simulink model "my_cstr"  (R2021b)
settings: Solver=ode45  StartTime=0.0  StopTime=1600  RelTol=1e-3
libraries: slpidlib x2
settings Model: PauseTimes=1  PacingRate=1000  Creator=Yi  LastModifiedBy=admin
settings DataIOCC: ReturnWorkspaceOutputs=off

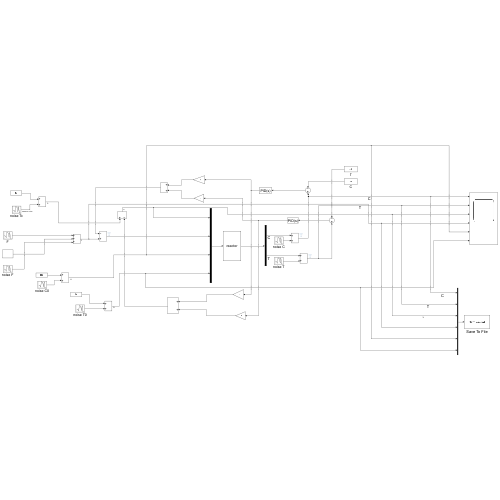
[thumbnail: Simulink's stored preview of the top-level diagram]
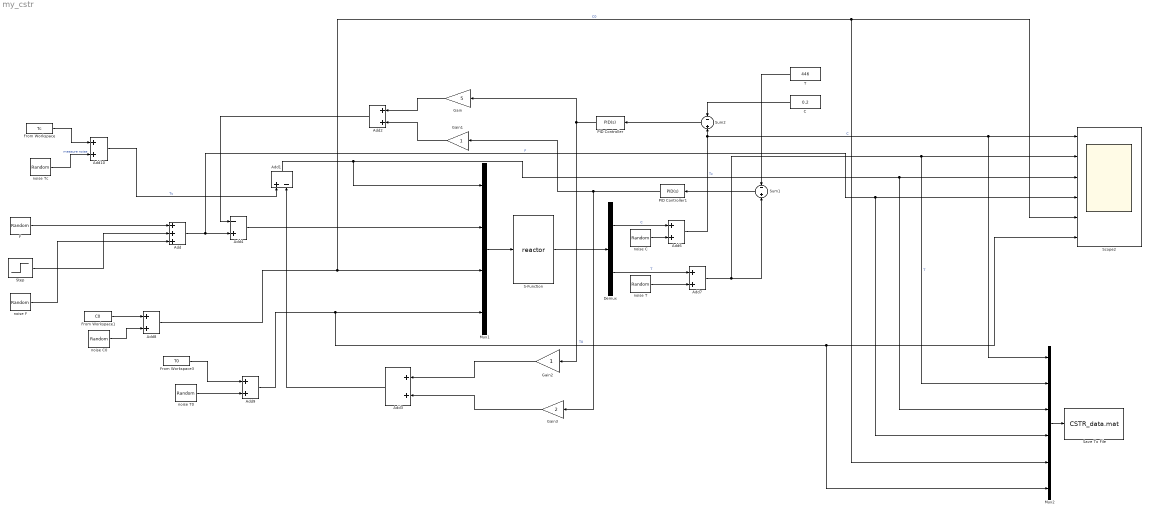
== system my_cstr ==
  Add : Sum  Inputs=+++
  Add1 : Sum  Inputs=+-
  Add{2..3,6..10} (7 alike) : Sum
  Add4 : Sum  Inputs=-+
  C : Constant  Value=0.2
  Demux : Demux  Outputs=2
  F : RandomNumber  Mean=100  Variance=30  SampleTime=1
  From Workspace : FromWorkspace  VariableName=Tc  SampleTime=1
  From Workspace1 : FromWorkspace  VariableName=C0  SampleTime=1
  From Workspace3 : FromWorkspace  VariableName=T0  SampleTime=1
  Gain : Gain  Gain=5
  Gain1 : Gain
  Gain2 : Gain
  Gain3 : Gain  Gain=2
  Mux1 : Mux
  Mux2 : Mux  Inputs=6
  PID Controller : slpidlib/PID Controller  Controller=PID  Form=Parallel  TimeDomain=Continuous-time  UseExternalTs=off  SampleTime=-1  IntegratorMethod=Forward Euler  FilterMethod=Forward Euler  ControllerParametersSource=internal  P=1  I=10  D=0.1  UseFilter=on  N=100  TunerSelectOption=Transfer Function Based (PID Tuner App)  InitialConditionSource=internal  InitialConditionForIntegrator=0  InitialConditionForFilter=0  DifferentiatorICPrevScaledInput=0  ExternalReset=none  TrackingMode=off  Kt=1  LimitOutput=off  SatLimitsSource=internal  UpperSaturationLimit=inf  LowerSaturationLimit=-inf  LinearizeAsGain=on  AntiWindupMode=none  Kb=1  POutMin=[]  POutMax=[]  IOutMin=[]  IOutMax=[]  DOutMin=[]  DOutMax=[]  NOutMin=[]  NOutMax=[]  SumOutMin=[]  SumOutMax=[]  SaturationOutMin=[]  SaturationOutMax=[]  PParamMin=[]  PParamMax=[]  IParamMin=[]  IParamMax=[]  DParamMin=[]  DParamMax=[]  NParamMin=[]  NParamMax=[]  KbParamMin=[]  KbParamMax=[]  KtParamMin=[]  KtParamMax=[]  KbOutMin=[]  KbOutMax=[]  KtOutMin=[]  KtOutMax=[]  IntegratorOutMin=[]  IntegratorOutMax=[]  FilterOutMin=[]  FilterOutMax=[]  SumI1OutMin=[]  SumI1OutMax=[]  SumI2OutMin=[]  SumI2OutMax=[]  SumI3OutMin=[]  SumI3OutMax=[]  SumI4OutMin=[]  SumI4OutMax=[]  SumDOutMin=[]  SumDOutMax=[]  DifferentiatorOutMin=[]  DifferentiatorOutMax=[]  FilterDiffOutCoefMin=[]  FilterDiffOutCoefMax=[]  ReciprocalOutMin=[]  ReciprocalOutMax=[]  SumDenOutMin=[]  SumDenOutMax=[]  SumNumOutMin=[]  SumNumOutMax=[]  DivideOutMin=[]  DivideOutMax=[]  UdiffTsProdOutMin=[]  UdiffTsProdOutMax=[]  NTsProdOutMin=[]  NTsProdOutMax=[]  UintegralTsProdOutMin=[]  UintegralTsProdOutMax=[]  UngainTsProdOutMin=[]  UngainTsProdOutMax=[]  IntegratorContinuousStateAttributes=''  IntegratorStateMustResolveToSignalObject=off  IntegratorRTWStateStorageClass=Auto  FilterContinuousStateAttributes=''  FilterStateMustResolveToSignalObject=off  FilterRTWStateStorageClass=Auto  ParallelPVariant=InternalParameters  IdealPVariant=Disabled  IVariant=InternalParameters  DVariant=InternalParameters  IntegratorVariant=Continuous  SatVariant=Disabled  AWVariant=Passthrough  PCopyVariant=Disabled  TRVariant=Disabled  FdbkBlocksVariant=Forward  IdealPFdbkVariant=Disabled  SatFdbkVariant=Disabled  DerivativeFilterVariant=ContFilter  NVariant=InternalParameters  NCopyVariant=Disabled  FilterICVariant=InternalICsFilter  IntegratorICVariant=InternalICs  ExternalResetVariant=Disabled  TRSumVariant=Passthrough  SumFdbkVariant=Disabled  SumVariant=Sum_PID  TsampFilterVariant=InternalTs  TsampNgainVariant=Passthrough  TsampIntegralVariant=Passthrough  ExternalSaturationOutDataTypeStr=Inherit: Same as second input
  PID Controller1 : slpidlib/PID Controller  Controller=PID  Form=Parallel  TimeDomain=Continuous-time  UseExternalTs=off  SampleTime=-1  IntegratorMethod=Forward Euler  FilterMethod=Forward Euler  ControllerParametersSource=internal  P=1  I=10  D=0.1  UseFilter=on  N=100  TunerSelectOption=Transfer Function Based (PID Tuner App)  InitialConditionSource=internal  InitialConditionForIntegrator=0  InitialConditionForFilter=0  DifferentiatorICPrevScaledInput=0  ExternalReset=none  TrackingMode=off  Kt=1  LimitOutput=off  SatLimitsSource=internal  UpperSaturationLimit=inf  LowerSaturationLimit=-inf  LinearizeAsGain=on  AntiWindupMode=none  Kb=1  POutMin=[]  POutMax=[]  IOutMin=[]  IOutMax=[]  DOutMin=[]  DOutMax=[]  NOutMin=[]  NOutMax=[]  SumOutMin=[]  SumOutMax=[]  SaturationOutMin=[]  SaturationOutMax=[]  PParamMin=[]  PParamMax=[]  IParamMin=[]  IParamMax=[]  DParamMin=[]  DParamMax=[]  NParamMin=[]  NParamMax=[]  KbParamMin=[]  KbParamMax=[]  KtParamMin=[]  KtParamMax=[]  KbOutMin=[]  KbOutMax=[]  KtOutMin=[]  KtOutMax=[]  IntegratorOutMin=[]  IntegratorOutMax=[]  FilterOutMin=[]  FilterOutMax=[]  SumI1OutMin=[]  SumI1OutMax=[]  SumI2OutMin=[]  SumI2OutMax=[]  SumI3OutMin=[]  SumI3OutMax=[]  SumI4OutMin=[]  SumI4OutMax=[]  SumDOutMin=[]  SumDOutMax=[]  DifferentiatorOutMin=[]  DifferentiatorOutMax=[]  FilterDiffOutCoefMin=[]  FilterDiffOutCoefMax=[]  ReciprocalOutMin=[]  ReciprocalOutMax=[]  SumDenOutMin=[]  SumDenOutMax=[]  SumNumOutMin=[]  SumNumOutMax=[]  DivideOutMin=[]  DivideOutMax=[]  UdiffTsProdOutMin=[]  UdiffTsProdOutMax=[]  NTsProdOutMin=[]  NTsProdOutMax=[]  UintegralTsProdOutMin=[]  UintegralTsProdOutMax=[]  UngainTsProdOutMin=[]  UngainTsProdOutMax=[]  IntegratorContinuousStateAttributes=''  IntegratorStateMustResolveToSignalObject=off  IntegratorRTWStateStorageClass=Auto  FilterContinuousStateAttributes=''  FilterStateMustResolveToSignalObject=off  FilterRTWStateStorageClass=Auto  ParallelPVariant=InternalParameters  IdealPVariant=Disabled  IVariant=InternalParameters  DVariant=InternalParameters  IntegratorVariant=Continuous  SatVariant=Disabled  AWVariant=Passthrough  PCopyVariant=Disabled  TRVariant=Disabled  FdbkBlocksVariant=Forward  IdealPFdbkVariant=Disabled  SatFdbkVariant=Disabled  DerivativeFilterVariant=ContFilter  NVariant=InternalParameters  NCopyVariant=Disabled  FilterICVariant=InternalICsFilter  IntegratorICVariant=InternalICs  ExternalResetVariant=Disabled  TRSumVariant=Passthrough  SumFdbkVariant=Disabled  SumVariant=Sum_PID  TsampFilterVariant=InternalTs  TsampNgainVariant=Passthrough  TsampIntegralVariant=Passthrough  ExternalSaturationOutDataTypeStr=Inherit: Same as second input
  S-Function : S-Function  FunctionName=reactor  SFunctionDeploymentMode=off  EnableBusSupport=off
  Save To File : ToFile  Filename=CSTR_data.mat  MatrixName=data  SampleTime=1
  Scope2 : Scope  NumInputPorts=6
  Step : Step  Time=1001  After=5  SampleTime=0
  Sum1 : Sum  Inputs=-+
  Sum2 : Sum  Inputs=-+
  T : Constant  Value=446
  noise C : RandomNumber  Variance=1e-5  SampleTime=1
  noise C0 : RandomNumber  Variance=1e-6  SampleTime=1
  noise F : RandomNumber  Variance=1e-6  SampleTime=1
  noise T : RandomNumber  Variance=0.005  SampleTime=1
  noise T0 : RandomNumber  Variance=1e-6  SampleTime=1
  noise Tc : RandomNumber  Variance=1e-6  SampleTime=1
  wires:
  Mux1/1 -> S-Function/1
  S-Function/1 -> Demux/1
  C/1 -> Sum2/1
  Sum2/1 -> PID Controller/1
  T/1 -> Sum1/1
  Sum1/1 -> PID Controller1/1
  PID Controller/1 -> Gain/1, Gain2/1
  PID Controller1/1 -> Gain3/1, Gain1/1
  Gain/1 -> Add2/1
  Gain1/1 -> Add2/2
  Gain2/1 -> Add3/1
  Gain3/1 -> Add3/2
  noise C/1 -> Add6/2
  Demux/1 -> Add6/1  "C"
  Add6/1 -> Mux2/1, Scope2/1, Sum2/2  "C"
  Demux/2 -> Add7/1  "T"
  noise T/1 -> Add7/2
  Add7/1 -> Mux2/2, Scope2/2, Sum1/2  "T"
  Add3/1 -> Add1/2
  noise C0/1 -> Add8/2
  Add8/1 -> Scope2/5, Mux2/5, Mux1/3  "C0"
  noise T0/1 -> Add9/2
  Add9/1 -> Mux2/6, Scope2/6, Mux1/4  "T0"
  Mux2/1 -> Save To File/1
  noise Tc/1 -> Add10/2  "measure noise"
  Add10/1 -> Add1/1  "Tc"
  Add1/1 -> Mux2/3, Scope2/3, Mux1/1  "Tc"
  F/1 -> Add/1
  Step/1 -> Add/2
  noise F/1 -> Add/3
  Add/1 -> Mux2/4, Scope2/4, Add4/2  "F"
  Add2/1 -> Add4/1
  Add4/1 -> Mux1/2
  From Workspace/1 -> Add10/1
  From Workspace1/1 -> Add8/1
  From Workspace3/1 -> Add9/1
